simulink model "inverter_1_phase"  (R2016a)
settings: Solver=VariableStepAuto  StartTime=0.0  StopTime=1  RelTol=1e-3
libraries: powerlib x26, simulink x1, powerlib_meascontrol x1
settings Model: Creator=Gorkem  LastModifiedBy=Gorkem

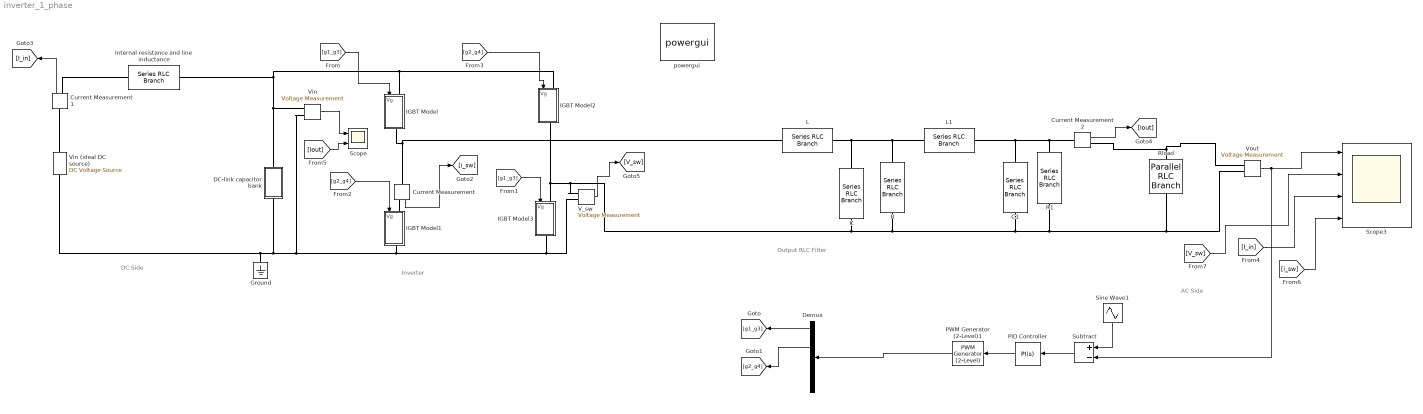
== system inverter_1_phase ==
  note: Inverter
  note: AC Side
  note: DC Side
  note: Output RLC Filter
  "      Internal resistance and line inductance" : powerlib/Elements/Series RLC Branch  LConnTagsString=__new0  RConnTagsString=__new0  BranchType=RL  Resistance=0.15  Inductance=5e-6  SetiL0=off  InitialCurrent=0  Capacitance=0  Setx0=off  InitialVoltage=0  Measurements=Branch voltage and current
  C : powerlib/Elements/Series RLC Branch  LConnTagsString=__new0  RConnTagsString=__new0  BranchType=RC  Resistance=0.5  Inductance=150e-6  SetiL0=off  InitialCurrent=0  Capacitance=150e-6  Setx0=off  InitialVoltage=0  Measurements=Branch voltage and current
  C1 : powerlib/Elements/Series RLC Branch  LConnTagsString=__new0  RConnTagsString=__new0  BranchType=RC  Resistance=0.5  Inductance=150e-6  SetiL0=off  InitialCurrent=0  Capacitance=150e-6  Setx0=off  InitialVoltage=0  Measurements=Branch voltage and current
  Current Measurement : powerlib/Measurements/Current Measurement  PhasorSimulation=off  OutputType=Complex  PSBequivalent=0
  Current Measurement1 : powerlib/Measurements/Current Measurement  PhasorSimulation=off  OutputType=Complex  PSBequivalent=0
  Current Measurement2 : powerlib/Measurements/Current Measurement  PhasorSimulation=off  OutputType=Complex  PSBequivalent=0
  "DC-link capacitor bank " : Subsystem
  Demux : Demux
  Ground : powerlib/Elements/Ground  LConnTagsString=a
  IGBT Model : Subsystem
  IGBT Model1 : Subsystem
  IGBT Model2 : Subsystem
  IGBT Model3 : Subsystem
  L : powerlib/Elements/Series RLC Branch  LConnTagsString=__new0  RConnTagsString=__new0  BranchType=RL  Resistance=0.2e-3  Inductance=30e-3  SetiL0=off  InitialCurrent=0  Capacitance=0  Setx0=off  InitialVoltage=0  Measurements=Branch voltage and current
  L1 : powerlib/Elements/Series RLC Branch  LConnTagsString=__new0  RConnTagsString=__new0  BranchType=RL  Resistance=0.2e-3  Inductance=30e-3  SetiL0=off  InitialCurrent=0  Capacitance=0  Setx0=off  InitialVoltage=0  Measurements=Branch voltage and current
  PID Controller : simulink/Continuous/PID Controller  Controller=PI  TimeDomain=Continuous-time  SampleTime=-1  IntegratorMethod=Forward Euler  FilterMethod=Forward Euler  Form=Parallel  UseFilter=on  ControllerParametersSource=internal  P=1  I=90  D=0  N=100  InitialConditionSource=internal  InitialConditionForIntegrator=0  InitialConditionForFilter=0  ExternalReset=none  LimitOutput=off  UpperSaturationLimit=inf  LowerSaturationLimit=-inf  LinearizeAsGain=on  AntiWindupMode=none  Kb=1  TrackingMode=off  Kt=1  PParamMin=[]  PParamMax=[]  IParamMin=[]  IParamMax=[]  DParamMin=[]  DParamMax=[]  NParamMin=[]  NParamMax=[]  KbParamMin=[]  KbParamMax=[]  KtParamMin=[]  KtParamMax=[]  POutMin=[]  POutMax=[]  IOutMin=[]  IOutMax=[]  DOutMin=[]  DOutMax=[]  NOutMin=[]  NOutMax=[]  KbOutMin=[]  KbOutMax=[]  KtOutMin=[]  KtOutMax=[]  IntegratorOutMin=[]  IntegratorOutMax=[]  FilterOutMin=[]  FilterOutMax=[]  SumOutMin=[]  SumOutMax=[]  SumI1OutMin=[]  SumI1OutMax=[]  SumI2OutMin=[]  SumI2OutMax=[]  SumI3OutMin=[]  SumI3OutMax=[]  SumDOutMin=[]  SumDOutMax=[]  SaturationOutMin=[]  SaturationOutMax=[]  IntegratorContinuousStateAttributes=''  IntegratorStateMustResolveToSignalObject=off  IntegratorRTWStateStorageClass=Auto  FilterContinuousStateAttributes=''  FilterStateMustResolveToSignalObject=off  FilterRTWStateStorageClass=Auto  DifferentiatorICPrevScaledInput=0  DifferentiatorOutMin=[]  DifferentiatorOutMax=[]
  PWM Generator (2-Level)1 : powerlib_meascontrol/Pulse & Signal Generators/PWM Generator (2-Level)  ModulatorType=Single-phase full-bridge (4 pulses)  ModulatorMode=Unsynchronized  Fc=1000  Pc=90  nF=20  MinMax="[ -8  8 ]"  SamplingTechnique=Natural  ModulatingSignals=off  m=0.8  Freq=50  Phase=0  Ts=0  ShowCarrierOutport=off
  R : powerlib/Elements/Series RLC Branch  LConnTagsString=__new0  RConnTagsString=__new0  BranchType=R  Resistance=8  Inductance=5e-6  SetiL0=off  InitialCurrent=0  Capacitance=0  Setx0=off  InitialVoltage=0  Measurements=Branch voltage and current
  R1 : powerlib/Elements/Series RLC Branch  LConnTagsString=__new0  RConnTagsString=__new0  BranchType=R  Resistance=8  Inductance=5e-6  SetiL0=off  InitialCurrent=0  Capacitance=0  Setx0=off  InitialVoltage=0  Measurements=Branch voltage and current
  Rload : powerlib/Elements/Parallel RLC Branch  LConnTagsString=a  RConnTagsString=__new0  BranchType=R  Resistance=250  Inductance=1e-3  SetiL0=off  InitialCurrent=0  Capacitance=1e-6  Setx0=off  InitialVoltage=0  Measurements=None
  Scope : Scope  NumInputPorts=2
  Scope3 : Scope  NumInputPorts=4
  Sine Wave1 : Sin  Amplitude=6.25  Frequency=2*pi*50  SampleTime=0
  Subtract : Sum  Inputs=+-
  V_sw : powerlib/Measurements/Voltage Measurement  PhasorSimulation=off  OutputType=Complex  PSBequivalent=0
  Vin : powerlib/Measurements/Voltage Measurement  PhasorSimulation=off  OutputType=Complex  PSBequivalent=0
  Vin (ideal DC source) : powerlib/Electrical Sources/DC Voltage Source  Amplitude=24  Measurements=Voltage
  Vout : powerlib/Measurements/Voltage Measurement  PhasorSimulation=off  OutputType=Complex  PSBequivalent=0
  powergui : powerlib/powergui  Priority=1  SimulationMode=Continuous  SolverType=Tustin/Backward Euler (TBE)  SampleTime=50e-6  frequency=60  SPID=off  DisableSnubberDevices=on  DisableRonSwitches=off  DisableVfSwitches=off  SwTol=0  DisplayEquations=off  Interpol=off  ExternalGateDelay=off  methode=off  Ts=10  FunctionMessages=on  echomessages=on  HookPort=off  EnableUseOfTLC=off  x0status=blocks  frequencyindice=0  Pbase=250  ErrMax=1e-4  Iterations=50  UnitsV=V  UnitsW=W  buscounter=0  RestoreLinks=warning  ResistiveCurrentMeasurement=off  Frange=[0:2:500]  Ylog=off  Xlog=on  ShowGrid=off  save=off  variable=ZData  structure=0  ZoomFFT=off  StartTime=0.0  cycles=1  DisplayStyle=1  fundamental=60  FreqAxis=off  MaxFrequency=1000  frequencyindicesteady=1  RmsSteady=1  display=off
  wires:
  [g1_g3] -> IGBT Model/1(Vg)
  [g1_g3] -> IGBT Model3/1(Vg)
  [g2_g4] -> IGBT Model1/1(Vg)
  [g2_g4] -> IGBT Model2/1(Vg)
  Vout/1 -> Subtract/2, Scope3/1
  [i_sw] -> Scope3/4
  Current Measurement1/1 -> [I_in]
  [V_sw] -> Scope3/2
  [I_in] -> Scope3/3
  Vin/1 -> Scope/1
  Current Measurement2/1 -> [Iout]
  [Iout] -> Scope/2
  V_sw/1 -> [V_sw]
  Current Measurement/1 -> [i_sw]
  Sine Wave1/1 -> Subtract/1
  Subtract/1 -> PID Controller/1
  PID Controller/1 -> PWM Generator (2-Level)1/1
  Demux/2 -> [g2_g4]
  Demux/1 -> [g1_g3]
  PWM Generator (2-Level)1/1 -> Demux/1
  connections:
  "DC-link capacitor bank "/LConn1 -- Vin/LConn1 -- "      Internal resistance and line inductance"/LConn1 -- IGBT Model2/LConn1 -- IGBT Model/LConn1
  Ground/LConn1 -- Vin (ideal DC source)/LConn1 -- "DC-link capacitor bank "/RConn1 -- V_sw/LConn2 -- IGBT Model3/RConn1 -- IGBT Model1/RConn1 -- Vin/LConn2
  Current Measurement1/LConn1 -- Vin (ideal DC source)/RConn1
  "      Internal resistance and line inductance"/RConn1 -- Current Measurement1/RConn1
  IGBT Model/RConn1 -- Current Measurement/LConn1 -- L/RConn1
  C/RConn1 -- L1/RConn1 -- R/RConn1 -- L/LConn1
  Rload/LConn1 -- Vout/LConn1 -- Current Measurement2/RConn1
  Current Measurement/RConn1 -- IGBT Model1/LConn1
  C1/RConn1 -- L1/LConn1 -- R1/RConn1 -- Current Measurement2/LConn1
  R/LConn1 -- C/LConn1 -- V_sw/LConn1 -- IGBT Model3/LConn1 -- IGBT Model2/RConn1 -- Rload/RConn1 -- Vout/LConn2 -- R1/LConn1 -- C1/LConn1

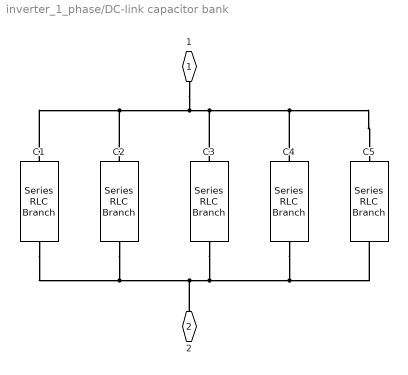
== system inverter_1_phase/DC-link capacitor bank  ==
  C1 : powerlib/Elements/Series RLC Branch  LConnTagsString=__new0  RConnTagsString=__new0  BranchType=RC  Resistance=8e-3  Inductance=680e-6  SetiL0=off  InitialCurrent=0  Capacitance=16e-3  Setx0=off  InitialVoltage=0  Measurements=Branch voltage and current
  "C2 " : powerlib/Elements/Series RLC Branch  LConnTagsString=__new0  RConnTagsString=__new0  BranchType=RC  Resistance=8e-3  Inductance=680e-6  SetiL0=off  InitialCurrent=0  Capacitance=16e-3  Setx0=off  InitialVoltage=0  Measurements=Branch voltage and current
  C3 : powerlib/Elements/Series RLC Branch  LConnTagsString=__new0  RConnTagsString=__new0  BranchType=RC  Resistance=8e-3  Inductance=680e-6  SetiL0=off  InitialCurrent=0  Capacitance=16e-3  Setx0=off  InitialVoltage=0  Measurements=Branch voltage and current
  C4 : powerlib/Elements/Series RLC Branch  LConnTagsString=__new0  RConnTagsString=__new0  BranchType=RC  Resistance=8e-3  Inductance=680e-6  SetiL0=off  InitialCurrent=0  Capacitance=16e-3  Setx0=off  InitialVoltage=0  Measurements=Branch voltage and current
  C5 : powerlib/Elements/Series RLC Branch  LConnTagsString=__new0  RConnTagsString=__new0  BranchType=RC  Resistance=8e-3  Inductance=680e-6  SetiL0=off  InitialCurrent=0  Capacitance=45e-3  Setx0=off  InitialVoltage=0  Measurements=Branch voltage and current
  1 : PMIOPort  Port=1  Side=Left
  2 : PMIOPort  Port=2  Side=Right
  connections:
  C1/LConn1 -- 1/RConn1 -- C3/LConn1 -- C4/LConn1 -- C5/LConn1 -- "C2 "/LConn1
  C1/RConn1 -- "C2 "/RConn1 -- 2/RConn1 -- C3/RConn1 -- C4/RConn1 -- C5/RConn1

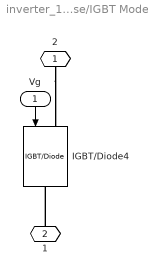
== system inverter_1_phase/IGBT Model ==
  Vg : Inport
  IGBT/Diode4 : powerlib/Power Electronics/IGBT//Diode  Ron=10e-3  Rs=20e-3  Cs=22e-6  Measurements=off
  2 : PMIOPort  Port=1  Side=Left
  1 : PMIOPort  Port=2  Side=Right
  wires:
  Vg/1 -> IGBT/Diode4/1
  connections:
  2/RConn1 -- IGBT/Diode4/LConn1
  1/RConn1 -- IGBT/Diode4/RConn1

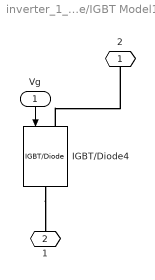
== system inverter_1_phase/IGBT Model1 ==
  Vg : Inport
  IGBT/Diode4 : powerlib/Power Electronics/IGBT//Diode  Ron=10e-3  Rs=20e-3  Cs=22e-6  Measurements=off
  2 : PMIOPort  Port=1  Side=Left
  1 : PMIOPort  Port=2  Side=Right
  wires:
  Vg/1 -> IGBT/Diode4/1
  connections:
  IGBT/Diode4/LConn1 -- 2/RConn1
  IGBT/Diode4/RConn1 -- 1/RConn1

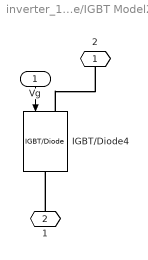
== system inverter_1_phase/IGBT Model2 ==
  Vg : Inport
  IGBT/Diode4 : powerlib/Power Electronics/IGBT//Diode  Ron=10e-3  Rs=20e-3  Cs=22e-6  Measurements=off
  2 : PMIOPort  Port=1  Side=Left
  1 : PMIOPort  Port=2  Side=Right
  wires:
  Vg/1 -> IGBT/Diode4/1
  connections:
  IGBT/Diode4/LConn1 -- 2/RConn1
  1/RConn1 -- IGBT/Diode4/RConn1

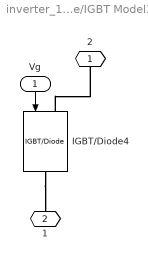
== system inverter_1_phase/IGBT Model3 ==
  Vg : Inport
  IGBT/Diode4 : powerlib/Power Electronics/IGBT//Diode  Ron=10e-3  Rs=20e-3  Cs=22e-6  Measurements=off
  2 : PMIOPort  Port=1  Side=Left
  1 : PMIOPort  Port=2  Side=Right
  wires:
  Vg/1 -> IGBT/Diode4/1
  connections:
  IGBT/Diode4/RConn1 -- 1/RConn1
  IGBT/Diode4/LConn1 -- 2/RConn1
